simulink model "Pendulum_LQ"  (R2021a)
settings: Solver=ode15s  StartTime=0.0  StopTime=100  RelTol=1e-3
undefined symbols (not defined in the file or in its folder): K_lqeta, K_lqx
settings Model: Creator=fabio  LastModifiedBy=fabio
settings SolverCC: AlgebraicLoopSolver=TrustRegion
settings OptimizationCC: BlockReduction=off  DefaultParameterBehavior=Inlined  BufferReuse=off
settings DebuggingCC: UnconnectedInputMsg=none  UnconnectedOutputMsg=none  UnconnectedLineMsg=none  SFMachineParentedDataDiag=warning

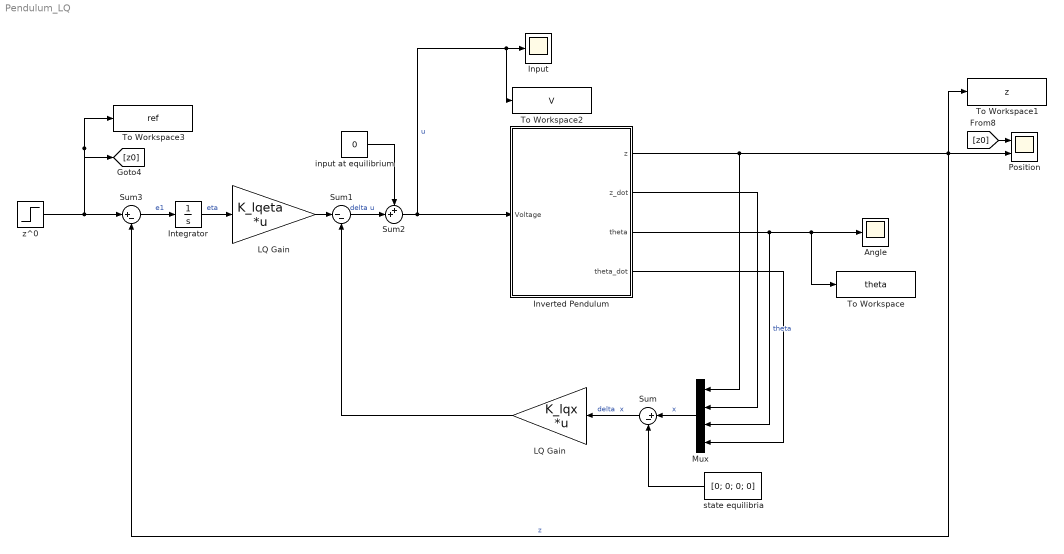
== system Pendulum_LQ ==
  Angle : Scope
  Input : Scope
  Integrator : Integrator
  Inverted Pendulum : Subsystem  mask(Inverted pendulum){MM=10, m=2, L=1, Rr=0.1, Ra=10, Kc=2, Ke=2, g=9.81, z0=0, theta0=0.2, z_dot0=0, theta_dot0=0, enableAnimation=on, animDt=0.075, wgn_var=[ 1e-5, 1e-6 ] * 0, exDistAmpl=0.3, enableSaturation=off}
      mask prompts: MM "Cart mass"; m "Damped mass"; L "Length"; Rr "Wheel radius"; Ra "Electric resistance"; g "Gravity"; z0 "Position"; theta0 "Orientation"; z_dot0 "Linear speed"; theta_dot0 "Angular speed"; enableAnimation "Show animation"; animDt "Animation time step"; wgn_var "y meas. noise variance"; exDistAmpl "Amplitude of perturbing force"; enableSaturation "Control saturation"
      mask help: Inverted pendulum nonlinear model, for the course of Advanced and Multivariable Control at Politecnico di Milano.
      mask DialogControl MM Tooltip: Mass of the cart [kg]
      mask DialogControl m Tooltip: Damped mass on the pendulum [kg]
      mask DialogControl L Tooltip: Length of the bar [m]
      mask DialogControl Rr Tooltip: Radius of the wheels [m]
      mask DialogControl Ra Tooltip: Resistance of the electric motor
      mask DialogControl Kc Tooltip: [V s/rad]
      mask DialogControl Ke Tooltip: [ Nm / A ]
      mask DialogControl g Tooltip: Gravity [m /s^2]
      mask DialogControl Container3 Prompt: Initial conditions
      mask DialogControl z0 Tooltip: Initial position of the cart [m]
      mask DialogControl theta0 Tooltip: Initial angle of the pendulum [rad]
      mask DialogControl z_dot0 Tooltip: Initial speed of the cart [m/s]
      mask DialogControl theta_dot0 Tooltip: Initial angular speed of the bar [rad/s]
      mask DialogControl Container4 Prompt: Animation
      mask DialogControl enableAnimation Tooltip: Show animations of the inverted pendulum
      mask DialogControl animDt Tooltip: Time step of the animation [s]
      mask DialogControl Container7 Prompt: Robustness
      mask DialogControl exDistAmpl Tooltip: Amplitude of the disturbance injected via the slider
      mask Display:
      | % Plot icon
      | plot([-10 10],[0 0],[-2 -2 2 2],[0 1 1 0],[0 3],[1 5]);
      | 
      | port_label('input', 1, 'V');
      | port_label('output', 1, 'z');
      | port_label('output', 2, 'z\_dot', 'interpreter', 'tex');
      | port_label('output', 3, '\theta', 'interpreter', 'tex');
      | port_label('output', 4, '\theta\_dot', 'interpreter', 'tex');
  LQ Gain : Gain  Gain=K_lqx  Multiplication=Matrix(K*u) (u vector)
  "LQ Gain " : Gain  Gain=K_lqeta  Multiplication=Matrix(K*u) (u vector)
  Mux : Mux
  Position : Scope  NumInputPorts=2
  Sum : Sum  Inputs=|+-
  Sum1 : Sum  Inputs=|--
  Sum2 : Sum  Inputs=++|
  Sum3 : Sum  Inputs=|+-
  To Workspace : ToWorkspace  VariableName=theta  SaveFormat=Timeseries  SampleTime=-1
  To Workspace1 : ToWorkspace  VariableName=z  SaveFormat=Timeseries  SampleTime=-1
  To Workspace2 : ToWorkspace  VariableName=V  SaveFormat=Timeseries  SampleTime=-1
  To Workspace3 : ToWorkspace  VariableName=ref  SaveFormat=Timeseries  SampleTime=-1
  input at equilibrium : Constant  Value=0
  "state equilibria " : Constant  Value=[0; 0; 0; 0]
  z^0 : Step  Time=25  After=0.25  SampleTime=0
  wires:
  Mux/1 -> Sum/1  "x"
  "state equilibria "/1 -> Sum/2
  LQ Gain/1 -> Sum1/2
  Sum1/1 -> Sum2/2  "delta u"
  input at equilibrium/1 -> Sum2/1
  "LQ Gain "/1 -> Sum1/1
  Integrator/1 -> "LQ Gain "/1  "eta"
  Sum3/1 -> Integrator/1  "e1"
  z^0/1 -> To Workspace3/1, [z0], Sum3/1
  Inverted Pendulum/4(theta_dot) -> Mux/4
  Inverted Pendulum/2(z_dot) -> Mux/2
  Sum/1 -> LQ Gain/1  "delta  x"
  Inverted Pendulum/1(z) -> Mux/1, Position/2, To Workspace1/1, Sum3/2  "z"
  Inverted Pendulum/3(theta) -> Mux/3, To Workspace/1, Angle/1  "theta"
  Sum2/1 -> Inverted Pendulum/1(Voltage), To Workspace2/1, Input/1  "u"
  [z0] -> Position/1

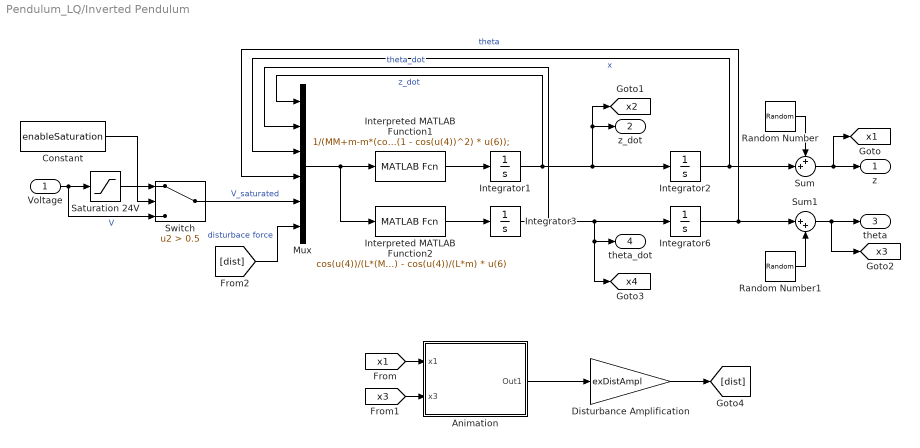
== system Pendulum_LQ/Inverted Pendulum ==
  Voltage : Inport
  Animation : Subsystem
  Constant : Constant  Value=enableSaturation
  Disturbance Amplification : Gain  Gain=exDistAmpl
  Integrator1 : Integrator  InitialCondition=z_dot0
  Integrator2 : Integrator  InitialCondition=z0
  Integrator3 : Integrator  InitialCondition=theta_dot0
  Integrator6 : Integrator  InitialCondition=theta0
  Interpreted MATLAB Function1 : MATLABFcn  MATLABFcn=1/(MM+m-m*(cos(u(4))^2)) * ( -Ke*Kc/(Ra*Rr^2) * u(1) - m*L*u(2)^2*sin(u(4)) + m*g*sin(u(4))*cos(u(4)) + Kc /(Ra*Rr) * u(5) + (1 - cos(u(4))^2) * u(6));  OutputDimensions=1
  Interpreted MATLAB Function2 : MATLABFcn  MATLABFcn=cos(u(4))/(L*(MM+m-m*(cos(u(4))^2))) * ( - Ke*Kc/(Ra*Rr^2) * u(1) - m*L*u(2)^2*sin(u(4)) + m*g*sin(u(4))*cos(u(4)) + Kc /(Ra*Rr) * u(5) + (1 - cos(u(4))^2) * u(6) ) + g/L * sin(u(4)) - cos(u(4))/(L*m) * u(6)  OutputDimensions=1
  Mux : Mux  Inputs=6
  Random Number : RandomNumber  Variance=wgn_var(1)  SampleTime=0.1
  Random Number1 : RandomNumber  Variance=wgn_var(2)  SampleTime=0.1
  Saturation 24V : Saturate  UpperLimit=24  LowerLimit=-24
  Sum : Sum  Inputs=++|
  Sum1 : Sum  Inputs=|++
  Switch : Switch  Criteria=u2 > Threshold  Threshold=0.5
  z : Outport
  z_dot : Outport  Port=2
  theta : Outport  Port=3
  theta_dot : Outport  Port=4
  tag scope: x1=global, x2=global, x3=global, x4=global
  wires:
  Animation/1(Out1) -> Disturbance Amplification/1
  Disturbance Amplification/1 -> [dist]
  [x1] -> Animation/1(x1)
  [x3] -> Animation/2(x3)
  Interpreted MATLAB Function1/1 -> Integrator1/1
  Integrator1/1 -> Mux/1, [x2], z_dot/1, Integrator2/1  "z_dot"
  [dist] -> Mux/6  "disturbace force"
  Integrator2/1 -> Sum/2, Mux/3  "x"
  Interpreted MATLAB Function2/1 -> Integrator3/1
  Integrator3/1 -> Mux/2, [x4], theta_dot/1, Integrator6/1  "theta_dot"
  Mux/1 -> Interpreted MATLAB Function2/1, Interpreted MATLAB Function1/1
  Integrator6/1 -> Sum1/1, Mux/4  "theta"
  Random Number1/1 -> Sum1/2
  Sum1/1 -> [x3], theta/1
  Random Number/1 -> Sum/1
  Sum/1 -> z/1, [x1]
  Voltage/1 -> Switch/3, Saturation 24V/1  "V"
  Constant/1 -> Switch/2
  Saturation 24V/1 -> Switch/1
  Switch/1 -> Mux/5  "V_saturated"

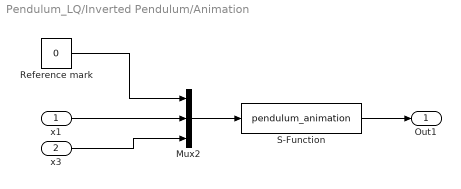
== system Pendulum_LQ/Inverted Pendulum/Animation ==
  x1 : Inport
  x3 : Inport  Port=2
  Mux2 : Mux  Inputs=3
  Reference mark : Constant  Value=0
  S-Function : S-Function  FunctionName=pendulum_animation  Parameters=[z0, theta0, L, enableAnimation, animDt]  SFunctionDeploymentMode=off  EnableBusSupport=off
  Out1 : Outport
  wires:
  Mux2/1 -> S-Function/1
  x3/1 -> Mux2/3
  Reference mark/1 -> Mux2/1
  x1/1 -> Mux2/2
  S-Function/1 -> Out1/1
